simulink model "simulaitons"  (Simulink 10.3)
settings: Solver=ode45  StartTime=0.0  StopTime=320  RelTol=1e-3  EnableMultiTasking=on
libraries: simulink x4
settings Model: Creator=xiaoling  LastModifiedBy=1179956468
settings SolverCC: AlgebraicLoopSolver=LineSearch
settings DataIOCC: LimitDataPoints=on  InspectSignalLogs=on
settings DebuggingCC: AlgebraicLoopMsg=none  SolverPrmCheckMsg=warning
settings GRTTargetCC: CombineOutputUpdateFcns=on  GRTInterface=off
settings ConfigComp: CovSFcnEnable=off

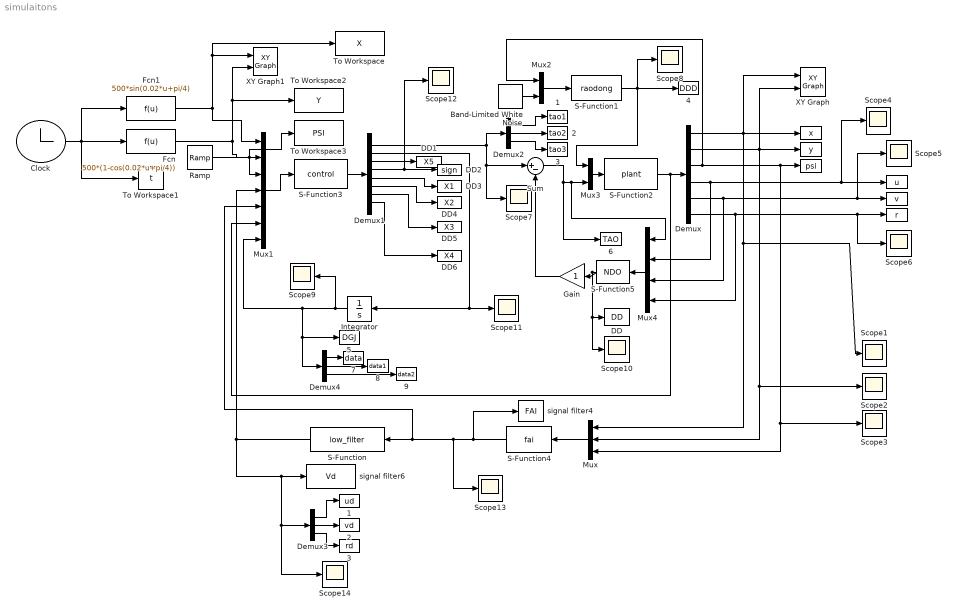
== system simulaitons ==
  " " : ToWorkspace  VariableName=x  SampleTime=-1
  "  " : ToWorkspace  VariableName=y  SampleTime=-1
  "   " : ToWorkspace  VariableName=psi  SampleTime=-1
  "    " : ToWorkspace  VariableName=u  SampleTime=-1
  "     " : ToWorkspace  VariableName=v  SampleTime=-1
  "      " : ToWorkspace  VariableName=r  SampleTime=-1
  "    1" : ToWorkspace  VariableName=ud  SampleTime=-1
  "    2" : ToWorkspace  VariableName=vd  SampleTime=-1
  "    3" : ToWorkspace  VariableName=rd  SampleTime=-1
  " 1" : ToWorkspace  VariableName=tao1  SampleTime=-1
  " 2" : ToWorkspace  VariableName=tao2  SampleTime=-1
  " 3" : ToWorkspace  VariableName=tao3  SampleTime=-1
  " 4" : ToWorkspace  VariableName=DDD  SampleTime=-1
  " 5" : ToWorkspace  VariableName=DGJ  SampleTime=-1
  " 6" : ToWorkspace  VariableName=TAO  SampleTime=-1
  " 7" : ToWorkspace  VariableName=data  SampleTime=-1
  " 8" : ToWorkspace  VariableName=data1  SampleTime=-1
  " 9" : ToWorkspace  VariableName=data2  SampleTime=-1
  Band-Limited White Noise : simulink/Sources/Band-Limited White Noise  Cov=[0.1]  Ts=0.1  seed=[23341]
  Clock : Clock
  DD : ToWorkspace  VariableName=DD  SampleTime=-1
  DD1 : ToWorkspace  VariableName=X5  SampleTime=-1
  DD2 : ToWorkspace  VariableName=sign  SampleTime=-1
  DD3 : ToWorkspace  VariableName=X1  SampleTime=-1
  DD4 : ToWorkspace  VariableName=X2  SampleTime=-1
  DD5 : ToWorkspace  VariableName=X3  SampleTime=-1
  DD6 : ToWorkspace  VariableName=X4  SampleTime=-1
  Demux : Demux  Outputs=6
  Demux1 : Demux  Outputs=8
  Demux2 : Demux  Outputs=3
  Demux3 : Demux  Outputs=3
  Demux4 : Demux  Outputs=3
  Fcn : Fcn  Expr=500*(1-cos(0.02*u+pi/4))
  Fcn1 : Fcn  Expr=500*sin(0.02*u+pi/4)
  Gain : Gain
  Integrator : Integrator
  Mux : Mux  Inputs=3
  Mux1 : Mux  Inputs=7
  Mux2 : Mux  Inputs=2
  Mux3 : Mux  Inputs=2
  Mux4 : Mux
  Ramp : simulink/Sources/Ramp  slope=0.01  start=0  InitialOutput=0
  S-Function : S-Function  FunctionName=low_filter  SFunctionDeploymentMode=off  EnableBusSupport=off
  S-Function1 : S-Function  FunctionName=raodong  SFunctionDeploymentMode=off  EnableBusSupport=off
  S-Function2 : S-Function  FunctionName=plant  SFunctionDeploymentMode=off  EnableBusSupport=off
  S-Function3 : S-Function  FunctionName=control  SFunctionDeploymentMode=off  EnableBusSupport=off
  S-Function4 : S-Function  FunctionName=fai  SFunctionDeploymentMode=off  EnableBusSupport=off
  S-Function5 : S-Function  FunctionName=NDO  SFunctionDeploymentMode=off  EnableBusSupport=off
  Scope{1..14} (14 alike) : Scope
  Sum : Sum  Inputs=|+-
  To Workspace : ToWorkspace  VariableName=X  SampleTime=-1
  To Workspace1 : ToWorkspace  VariableName=t  SampleTime=-1
  To Workspace2 : ToWorkspace  VariableName=Y  SampleTime=-1
  To Workspace3 : ToWorkspace  VariableName=PSI  SampleTime=-1
  XY Graph : simulink/Sinks/XY Graph  xmin=-500  xmax=500  ymin=0  ymax=1000  st=-1
  XY Graph1 : simulink/Sinks/XY Graph  xmin=-500  xmax=500  ymin=0  ymax=1000  st=-1
  signal filter4 : ToWorkspace  VariableName=FAI  SampleTime=-1
  signal filter6 : ToWorkspace  VariableName=Vd  SampleTime=-1
  wires:
  Mux1/1 -> S-Function3/1
  S-Function4/1 -> signal filter4/1, S-Function/1, Mux1/5, Scope13/1
  S-Function2/1 -> Mux1/6, Demux/1
  S-Function/1 -> Mux1/4, signal filter6/1, Scope14/1, Demux3/1
  Demux/1 -> " "/1, Mux/1, Scope1/1, XY Graph/1
  Demux/2 -> "  "/1, Mux/2, Scope2/1, XY Graph/2
  Demux/3 -> "   "/1, Mux/3, Scope3/1, Mux2/1
  Demux/4 -> "    "/1, Scope4/1, Mux4/2
  Demux/5 -> "     "/1, Scope5/1, Mux4/3
  Demux/6 -> "      "/1, Scope6/1, Mux4/4
  Mux/1 -> S-Function4/1
  S-Function3/1 -> Demux1/1
  Fcn1/1 -> Mux1/1, XY Graph1/1, To Workspace/1
  Clock/1 -> Fcn/1, To Workspace1/1, Fcn1/1
  Ramp/1 -> Mux1/3, To Workspace3/1
  Demux2/1 -> " 1"/1
  Demux2/2 -> " 2"/1
  Demux2/3 -> " 3"/1
  Fcn/1 -> Mux1/2, XY Graph1/2, To Workspace2/1
  Mux3/1 -> S-Function2/1
  Band-Limited White Noise/1 -> Mux2/2
  Mux2/1 -> S-Function1/1
  S-Function1/1 -> Mux3/1, Scope8/1, " 4"/1
  Demux1/1 -> Scope7/1, Sum/1, Demux2/1
  Integrator/1 -> Scope9/1, Demux4/1, " 5"/1, Mux1/7
  Demux4/1 -> " 7"/1
  Demux4/2 -> " 8"/1
  Demux4/3 -> " 9"/1
  Demux1/2 -> Integrator/1, Scope11/1
  Sum/1 -> Mux4/1, Mux3/2, " 6"/1
  Mux4/1 -> S-Function5/1
  S-Function5/1 -> Scope10/1, DD/1, Gain/1
  Gain/1 -> Sum/2
  Demux1/3 -> DD1/1
  Demux1/4 -> DD2/1, Scope12/1
  Demux1/6 -> DD4/1
  Demux1/7 -> DD5/1
  Demux1/8 -> DD6/1
  Demux1/5 -> DD3/1
  Demux3/1 -> "    1"/1
  Demux3/2 -> "    2"/1
  Demux3/3 -> "    3"/1
